simulink model "RT_ueb3_2g12"  (R2013a)
settings: Solver=ode45  StartTime=0.0  StopTime=10.0  RelTol=1e-3
values from neighbouring files (symbols this model uses):
  k = 1    [RT_Klausur_SS2014.m]    (also in RT_ctrl_analyse_proc.m = 5; RT_dennis_draussen.m = 50; RT_klausurvorb.m = 0.2; RT_lab_paramLead.m)
settings Model: Creator=mainster  LastModifiedBy=mainster

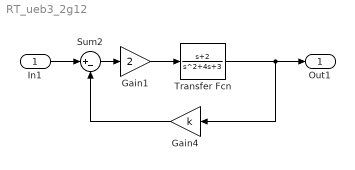
== system RT_ueb3_2g12 ==
  In1 : Inport
  Gain1 : Gain  Gain=2
  Gain4 : Gain  Gain=k
  Sum2 : Sum  Inputs=|+-
  Transfer Fcn : TransferFcn  Numerator=[1 2]  Denominator=[1 4 3]
  Out1 : Outport
  wires:
  Sum2/1 -> Gain1/1
  Gain4/1 -> Sum2/2
  Transfer Fcn/1 -> Out1/1, Gain4/1
  In1/1 -> Sum2/1
  Gain1/1 -> Transfer Fcn/1
